simulink model "myOneInOneOut"  (R2024a)
settings: Solver=VariableStepAuto  StartTime=0.0  StopTime=10.0  RelTol=1e-3
InitFcn:
  | close all;
  | clear all;
  | % Excelファイルのパスとファイル名
  | [file, path] = uigetfile('*.xlsx', 'Excelファイルを選択してください');
  | if isequal(file, 0)
  |     disp('ファイルが選択されませんでした。');
  |     return;
  | else
  |     filepath = fullfile(path, file);
  | end
  | % シート名またはシートインデックス
  | sheet = 'Sheet1'; % シート名を指定する場合
  | % sheet = 1; % シートインデックスを指定する場合
  | % Excelファイルからデータを読み込む
  | data = readcell(filepath, 'Sheet', sheet);
  | x1 = cellfun(@double, data(2:end, 1));
StopFcn:
  | y = out.y.Data;
  | figure;
  | scatter(x1(y == -1), y(y == -1), 'filled', 'b'); % yが-1の点をでプロット
  | hold on
  | scatter(x1(y == 1), y(y == 1), 'filled', 'r'); % yが1の点を赤でプロット
  | grid on
settings Model: Creator=mashi  LastModifiedBy=mashi

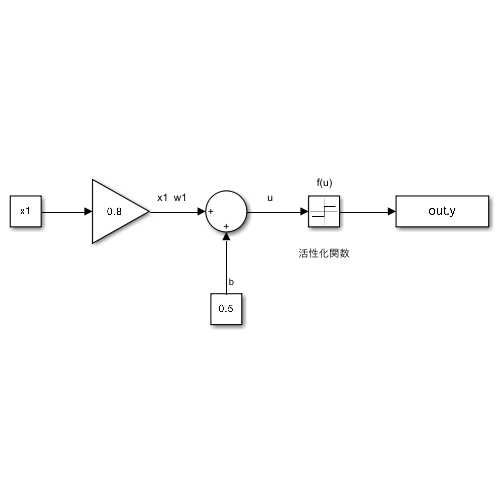
[thumbnail: Simulink's stored preview of the top-level diagram]
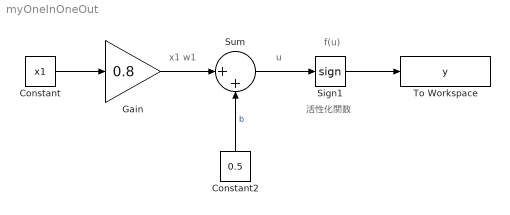
== system myOneInOneOut ==
  note: 活性化関数
  note: u
  note: f(u)
  note: x1 w1
  Constant : Constant  Value=x1
  Constant2 : Constant  Value=0.5
  Gain : Gain  Gain=0.8
  Sign1 : Signum
  Sum : Sum  Inputs=|++
  To Workspace : ToWorkspace  VariableName=y  SaveFormat=Timeseries  SampleTime=-1
  wires:
  Constant/1 -> Gain/1
  Gain/1 -> Sum/1
  Sign1/1 -> To Workspace/1
  Sum/1 -> Sign1/1
  Constant2/1 -> Sum/2  "b"
